simulink model "model_no_linear_observador"  (R2022a)
settings: Solver=VariableStepAuto  StartTime=0  StopTime=100  RelTol=1e-3
values from neighbouring files (symbols this model uses):
  A = [ 0 1 0  0 ... (first row only)    [ball_and_beam_pfc.m]
  amplitude_entrada = 0.05    [ball_and_beam_pfc.m]
  B = [0 ... (first row only)    [ball_and_beam_pfc.m]
  bool_degrau = 1    [ball_and_beam_pfc.m]
  C = [0 0 1 0]    [ball_and_beam_pfc.m]
  g = 9.8    [ball_and_beam_pfc.m]    (also in nonlinear_ball_and_beam.m)
  Jv = (1/2) * mv * L^2    (= 0.058703125)    [ball_and_beam_pfc.m]    (also in nonlinear_ball_and_beam.m)
  k_seguimento = K_nulo(1:4)    [ball_and_beam_pfc.m]
  ki_seguimento = K_nulo(5)    [ball_and_beam_pfc.m]
  L = 0.425    [ball_and_beam_pfc.m]    (also in nonlinear_ball_and_beam.m)
  L_observer_lqr = L_observador_lqr'    [ball_and_beam_pfc.m]
  mb = 0.064    [ball_and_beam_pfc.m]    (also in nonlinear_ball_and_beam.m)
  mv = 0.65    [ball_and_beam_pfc.m]    (also in nonlinear_ball_and_beam.m)
libraries: vrlib x3
settings Model: Creator=Notebook_Artur  LastModifiedBy=Notebook_Artur

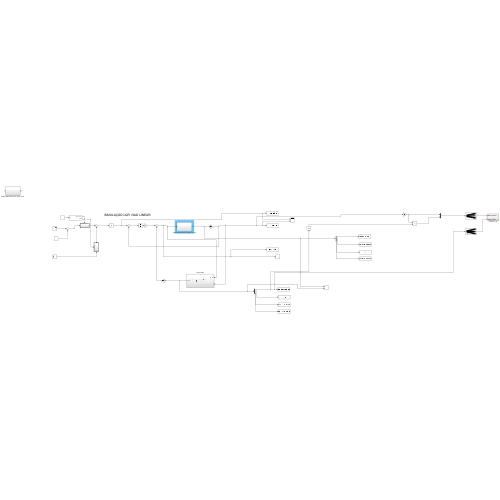
[thumbnail: Simulink's stored preview of the top-level diagram]
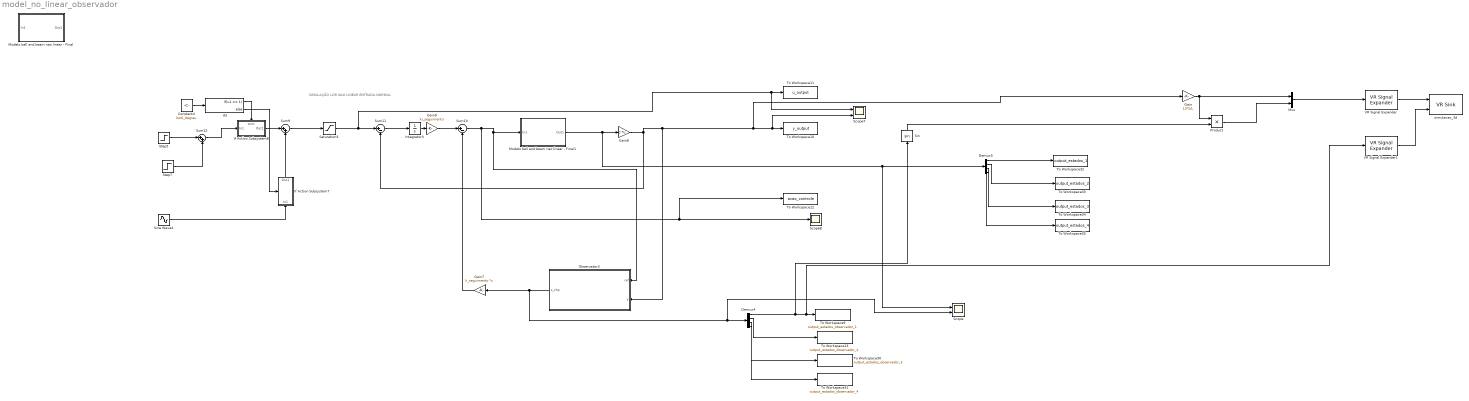
== system model_no_linear_observador ==
  note: SIMULAÇÃO LQR NAO LINEAR ENTRADA NORMAL
  Constant4 : Constant  Value=bool_degrau
  Demux4 : Demux
  Demux5 : Demux
  Gain : Gain  Gain=13*2/L
  Gain7 : Gain  Gain=k_seguimento  Multiplication=Matrix(K*u)
  Gain8 : Gain  Gain=C  Multiplication=Matrix(K*u)
  Gain9 : Gain  Gain=ki_seguimento
  If Action Subsystem7 : Subsystem  TreatAsAtomicUnit=on
  If Action Subsystem8 : Subsystem  TreatAsAtomicUnit=on
  If3 : If  IfExpression=u1 == 1
  Integrator3 : Integrator
  Modelo ball and beam nao linear - Final : Subsystem
  Modelo ball and beam nao linear - Final1 : Subsystem
  Mux : Mux  Inputs=2
  Observador3 : Subsystem
  Product : Product
  Saturation3 : Saturate  UpperLimit=L/2  LowerLimit=-L/2
  Scope : Scope  NumInputPorts=2
  Scope7 : Scope  NumInputPorts=2
  Scope8 : Scope
  Sin : Trigonometry
  Sine Wave4 : Sin  Amplitude=amplitude_entrada  Frequency=0.1  SampleTime=0
  Step5 : Step  After=amplitude_entrada  SampleTime=0
  Step7 : Step  Time=100  After=-2*amplitude_entrada  SampleTime=0
  Sum10 : Sum  Inputs=|+-
  Sum11 : Sum  Inputs=|+-
  Sum12 : Sum  Inputs=|++
  Sum9 : Sum  Inputs=|++
  To Workspace10 : ToWorkspace  VariableName=y_output  SaveFormat=Timeseries  SampleTime=-1
  To Workspace11 : ToWorkspace  VariableName=u_output  SaveFormat=Timeseries  SampleTime=-1
  To Workspace12 : ToWorkspace  VariableName=acao_controle  SaveFormat=Timeseries  SampleTime=-1
  To Workspace13 : ToWorkspace  VariableName=output_estados_observador_2  SaveFormat=Timeseries  SampleTime=-1
  To Workspace30 : ToWorkspace  VariableName=output_estados_observador_3  SaveFormat=Timeseries  SampleTime=-1
  To Workspace31 : ToWorkspace  VariableName=output_estados_observador_4  SaveFormat=Timeseries  SampleTime=-1
  To Workspace32 : ToWorkspace  VariableName=output_estados_1  SaveFormat=Timeseries  SampleTime=-1
  To Workspace33 : ToWorkspace  VariableName=output_estados_2  SaveFormat=Timeseries  SampleTime=-1
  To Workspace34 : ToWorkspace  VariableName=output_estados_3  SaveFormat=Timeseries  SampleTime=-1
  To Workspace35 : ToWorkspace  VariableName=output_estados_4  SaveFormat=Timeseries  SampleTime=-1
  To Workspace9 : ToWorkspace  VariableName=output_estados_observador_1  SaveFormat=Timeseries  SampleTime=-1
  VR Signal Expander : vrlib/VR Signal Expander  outwidth=3  outidx=[1 3]
  VR Signal Expander1 : vrlib/VR Signal Expander  outwidth=4  outidx=[4]
  simulacao_3d : vrlib/VR Sink  InstantiateOnLoad=on  SampleTime=0.1  ViewEnable=on  RemoteChange=off  RemoteView=off  FieldsWritten=Ball.translation.3.1.1.double#beam.rotation.4.1.1.double  WorldFileName=3d_ball_and_beam4.x3d  AutoView=on  VideoDimensions=[]  AllowVariableSize=off
  wires:
  Demux5/3 -> To Workspace34/1
  Demux5/2 -> To Workspace33/1
  Demux4/2 -> To Workspace13/1
  Demux4/3 -> To Workspace30/1
  Sum11/1 -> Integrator3/1
  Saturation3/1 -> To Workspace11/1, Scope7/1, Sum11/1
  Gain7/1 -> Sum10/2
  Observador3/1(x_chp) -> Scope/2, Demux4/1, Gain7/1
  Gain8/1 -> Gain/1, Scope7/2, To Workspace10/1, Observador3/2(y), Sum11/2
  Demux5/1 -> To Workspace32/1
  If Action Subsystem8/1(Out1) -> Sum9/1
  Sine Wave4/1 -> If Action Subsystem7/1(In1)
  Demux4/4 -> To Workspace31/1
  Modelo ball and beam nao linear - Final1/1(Out1) -> Scope/1, Demux5/1, Gain8/1
  Step7/1 -> Sum12/2
  If Action Subsystem7/1(Out1) -> Sum9/2
  Demux5/4 -> To Workspace35/1
  Sum10/1 -> To Workspace12/1, Scope8/1, Modelo ball and beam nao linear - Final1/1(In1), Observador3/1(ref)
  Constant4/1 -> If3/1
  Step5/1 -> Sum12/1
  Sum12/1 -> If Action Subsystem8/1(In1)
  Sum9/1 -> Saturation3/1
  Gain9/1 -> Sum10/1
  If3/1 -> If Action Subsystem8/Action
  Integrator3/1 -> Gain9/1
  If3/2 -> If Action Subsystem7/Action
  Demux4/1 -> Sin/1, VR Signal Expander1/1, To Workspace9/1
  VR Signal Expander/1 -> simulacao_3d/1
  VR Signal Expander1/1 -> simulacao_3d/2
  Product/1 -> Mux/2
  Gain/1 -> Product/1, Mux/1
  Mux/1 -> VR Signal Expander/1
  Sin/1 -> Product/2

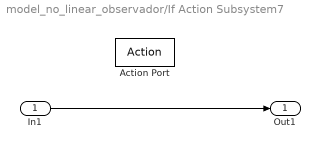
== system model_no_linear_observador/If Action Subsystem7 ==
  In1 : Inport
  Action Port : ActionPort  ActionPortLabel=else
  Out1 : Outport
  wires:
  In1/1 -> Out1/1

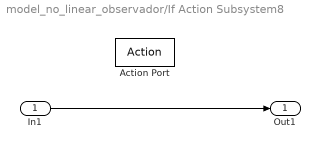
== system model_no_linear_observador/If Action Subsystem8 ==
  In1 : Inport
  Action Port : ActionPort  ActionPortLabel=if(u1 == 1)
  Out1 : Outport
  wires:
  In1/1 -> Out1/1

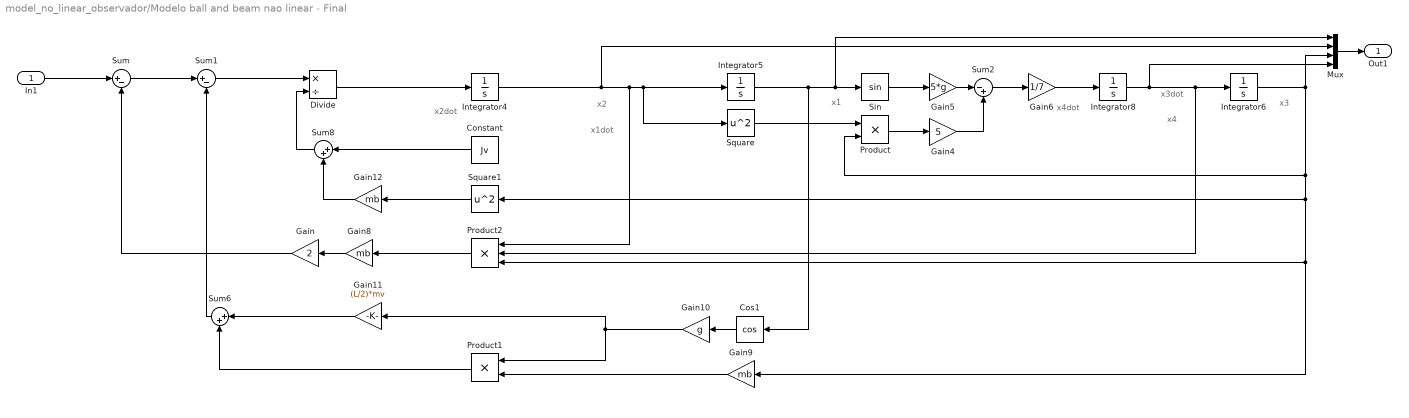
== system model_no_linear_observador/Modelo ball and beam nao linear - Final ==
  note: x3
  note: x3dot
  note: x4
  note: x4dot
  note: x1
  note: x1dot
  note: x2dot
  note: x2
  In1 : Inport
  Constant : Constant  Value=Jv
  Cos1 : Trigonometry  Operator=cos
  Divide : Product  Inputs=*/
  Gain : Gain  Gain=2
  Gain10 : Gain  Gain=g
  Gain11 : Gain  Gain=(L/2)*mv
  Gain12 : Gain  Gain=mb
  Gain4 : Gain  Gain=5
  Gain5 : Gain  Gain=5*g
  Gain6 : Gain  Gain=1/7
  Gain8 : Gain  Gain=mb
  Gain9 : Gain  Gain=mb
  Integrator{4..6,8} (4 alike) : Integrator
  Mux : Mux
  Product : Product
  Product1 : Product
  Product2 : Product  Inputs=3
  Sin : Trigonometry
  Square : Math  Operator=square
  Square1 : Math  Operator=square
  Sum : Sum  Inputs=|+-
  Sum1 : Sum  Inputs=|+-
  Sum2 : Sum  Inputs=|-+
  Sum6 : Sum  Inputs=|++
  Sum8 : Sum  Inputs=|++
  Out1 : Outport
  wires:
  Integrator8/1 -> Mux/4, Product2/2, Integrator6/1
  Integrator5/1 -> Sin/1, Mux/1, Cos1/1
  Sum6/1 -> Sum1/2
  Sum2/1 -> Gain6/1
  Gain10/1 -> Product1/1, Gain11/1
  Square/1 -> Product/1
  Integrator6/1 -> Mux/3, Gain9/1, Product2/3, Square1/1, Product/2
  Gain11/1 -> Sum6/1
  Gain12/1 -> Sum8/2
  Gain6/1 -> Integrator8/1
  Gain4/1 -> Sum2/2
  Gain9/1 -> Product1/2
  Cos1/1 -> Gain10/1
  Divide/1 -> Integrator4/1
  Product2/1 -> Gain8/1
  Product/1 -> Gain4/1
  Square1/1 -> Gain12/1
  Sum8/1 -> Divide/2
  Product1/1 -> Sum6/2
  Constant/1 -> Sum8/1
  Mux/1 -> Out1/1
  Gain5/1 -> Sum2/1
  Sin/1 -> Gain5/1
  Gain8/1 -> Gain/1
  Sum1/1 -> Divide/1
  Sum/1 -> Sum1/1
  Integrator4/1 -> Mux/2, Product2/1, Square/1, Integrator5/1
  In1/1 -> Sum/1
  Gain/1 -> Sum/2

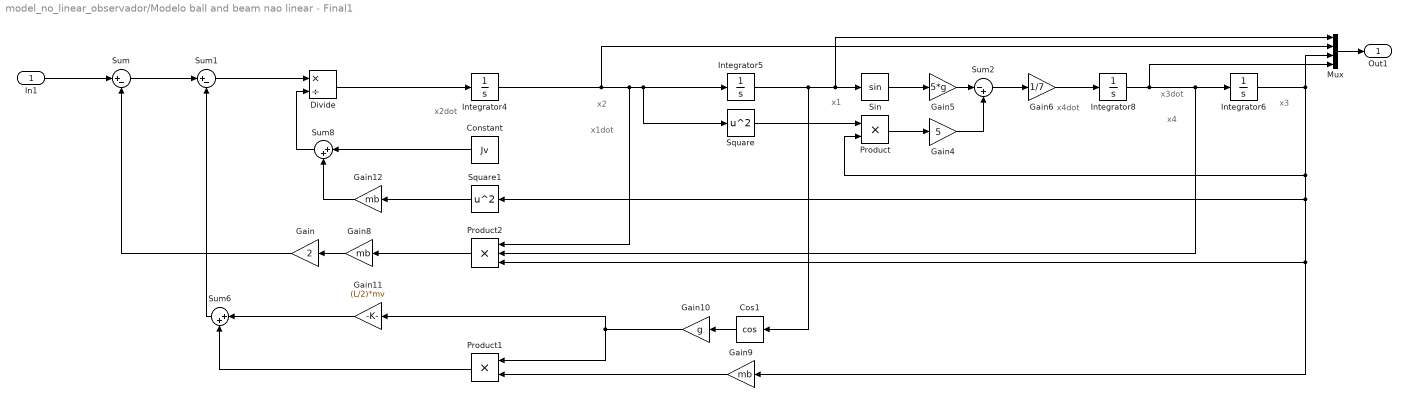
== system model_no_linear_observador/Modelo ball and beam nao linear - Final1 ==
  note: x3
  note: x3dot
  note: x4
  note: x4dot
  note: x1
  note: x1dot
  note: x2dot
  note: x2
  In1 : Inport
  Constant : Constant  Value=Jv
  Cos1 : Trigonometry  Operator=cos
  Divide : Product  Inputs=*/
  Gain : Gain  Gain=2
  Gain10 : Gain  Gain=g
  Gain11 : Gain  Gain=(L/2)*mv
  Gain12 : Gain  Gain=mb
  Gain4 : Gain  Gain=5
  Gain5 : Gain  Gain=5*g
  Gain6 : Gain  Gain=1/7
  Gain8 : Gain  Gain=mb
  Gain9 : Gain  Gain=mb
  Integrator{4..6,8} (4 alike) : Integrator
  Mux : Mux
  Product : Product
  Product1 : Product
  Product2 : Product  Inputs=3
  Sin : Trigonometry
  Square : Math  Operator=square
  Square1 : Math  Operator=square
  Sum : Sum  Inputs=|+-
  Sum1 : Sum  Inputs=|+-
  Sum2 : Sum  Inputs=|-+
  Sum6 : Sum  Inputs=|++
  Sum8 : Sum  Inputs=|++
  Out1 : Outport
  wires:
  Integrator8/1 -> Mux/4, Product2/2, Integrator6/1
  Integrator5/1 -> Sin/1, Mux/1, Cos1/1
  Sum6/1 -> Sum1/2
  Sum2/1 -> Gain6/1
  Gain10/1 -> Product1/1, Gain11/1
  Square/1 -> Product/1
  Integrator6/1 -> Mux/3, Gain9/1, Product2/3, Square1/1, Product/2
  Gain11/1 -> Sum6/1
  Gain12/1 -> Sum8/2
  Gain6/1 -> Integrator8/1
  Gain4/1 -> Sum2/2
  Gain9/1 -> Product1/2
  Cos1/1 -> Gain10/1
  Divide/1 -> Integrator4/1
  Product2/1 -> Gain8/1
  Product/1 -> Gain4/1
  Square1/1 -> Gain12/1
  Sum8/1 -> Divide/2
  Product1/1 -> Sum6/2
  Constant/1 -> Sum8/1
  Mux/1 -> Out1/1
  Gain5/1 -> Sum2/1
  Sin/1 -> Gain5/1
  Gain8/1 -> Gain/1
  Sum1/1 -> Divide/1
  Sum/1 -> Sum1/1
  Integrator4/1 -> Mux/2, Product2/1, Square/1, Integrator5/1
  In1/1 -> Sum/1
  Gain/1 -> Sum/2

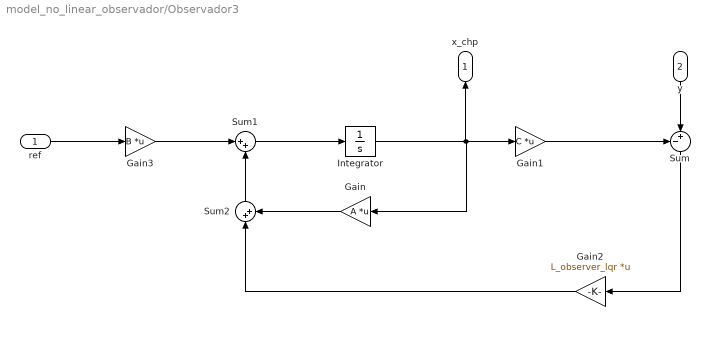
== system model_no_linear_observador/Observador3 ==
  ref : Inport
  y : Inport  Port=2
  Gain : Gain  Gain=A  Multiplication=Matrix(K*u)
  Gain1 : Gain  Gain=C  Multiplication=Matrix(K*u)
  Gain2 : Gain  Gain=L_observer_lqr  Multiplication=Matrix(K*u)
  Gain3 : Gain  Gain=B  Multiplication=Matrix(K*u)
  Integrator : Integrator
  Sum : Sum  Inputs=-+|
  Sum1 : Sum  Inputs=|++
  Sum2 : Sum  Inputs=|++
  x_chp : Outport
  wires:
  Integrator/1 -> x_chp/1, Gain1/1, Gain/1
  Sum/1 -> Gain2/1
  Gain1/1 -> Sum/1
  Gain/1 -> Sum2/2
  y/1 -> Sum/2
  Sum2/1 -> Sum1/2
  Gain2/1 -> Sum2/1
  Sum1/1 -> Integrator/1
  ref/1 -> Gain3/1
  Gain3/1 -> Sum1/1
